simulink model "wec_reinforcementlearning"  (R2017b)
settings: Solver=VariableStepAuto  StartTime=0.0  StopTime=900  RelTol=1e-3
values from neighbouring files (symbols this model uses):
  B = zeros(vz,hz)    [ACTOR_CRITIC & SARSA.m]    (also in InputDataExtraction.m = 0.01; TDlearningExampleEforPosting.m)
  K = K_stiff*133333    (= 199999.5)    [InputDataExtraction.m]
  m = min(Out,[],2)    [ContinousControl.m]    (also in RL.m; RealTime_modif22.m)
undefined symbols (not defined in the file or in its folder): A, dzb_0, wp, zb_0
settings Model: Creator=brekken  LastModifiedBy=brekken
settings CodeAppCC: StateflowObjectComments=on

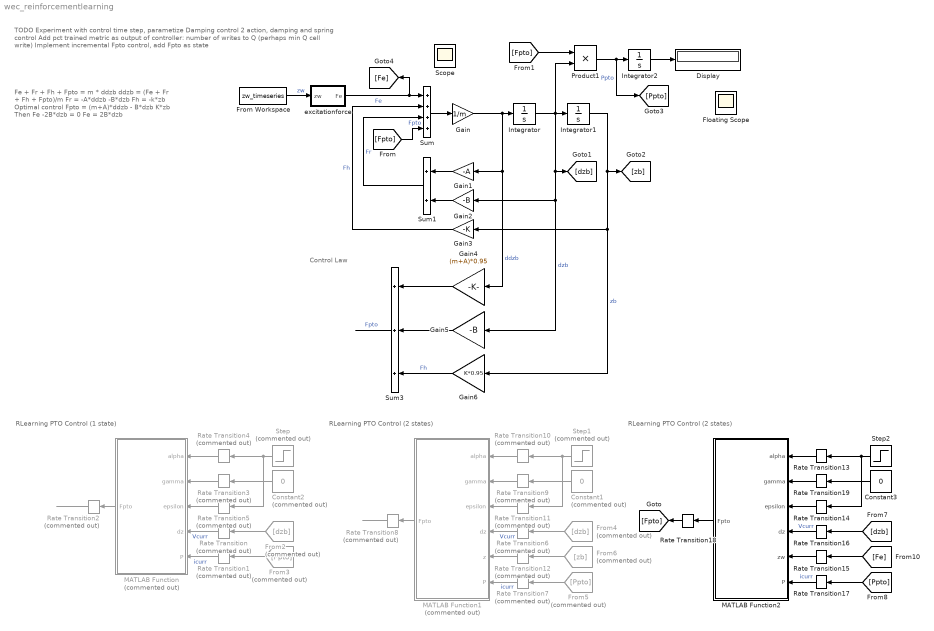
== system wec_reinforcementlearning ==
  note: Control Law
  note: TODO
      |
      | Experiment with control time step, parametize
      | Damping control
      | 2 action, damping and spring control
      | Add pct trained metric as output of controller: number of writes to Q (perhaps min Q cell write)
      | Implement incremental Fpto control, add Fpto as state
  note: RLearning PTO Control (1 state)
  note: Fe + Fr + Fh + Fpto = m * ddzb
      | ddzb = (Fe + Fr + Fh + Fpto)/m
      |
      | Fr = -A*ddzb -B*dzb
      |
      | Fh = -k*zb
      |
      | Optimal control
      | Fpto = (m+A)*ddzb - B*dzb K*zb
      | Then
      | Fe -2B*dzb = 0
      | Fe = 2B*dzb
  note: RLearning PTO Control (2 states)
  note: RLearning PTO Control (2 states)
  Constant1 : Constant  Commented=on  Value=0
  Constant2 : Constant  Commented=on  Value=0
  Constant3 : Constant  Value=0
  Display : Display
  Floating Scope : Scope
      settings: Floating=on
  From Workspace : FromWorkspace  VariableName=zw_timeseries  SampleTime=0  OutputAfterFinalValue=Setting to zero
  From2 : From  Commented=on  GotoTag=dzb
  From3 : From  Commented=on  GotoTag=Ppto
  From4 : From  Commented=on  GotoTag=dzb
  From5 : From  Commented=on  GotoTag=Ppto
  From6 : From  Commented=on  GotoTag=zb
  Gain : Gain  Gain=1/m
  Gain1 : Gain  Gain=-A
  Gain2 : Gain  Gain=-B
  Gain3 : Gain  Gain=-K
  Gain4 : Gain  Gain=(m+A)*0.95
  Gain5 : Gain  Gain=-B
  Gain6 : Gain  Gain=K*0.95
  Integrator : Integrator  InitialCondition=dzb_0
  Integrator1 : Integrator  InitialCondition=zb_0
  Integrator2 : Integrator
  MATLAB Function : MATLAB Function  Commented=on  TreatAsAtomicUnit=on
  MATLAB Function1 : MATLAB Function  Commented=on  TreatAsAtomicUnit=on
  MATLAB Function2 : MATLAB Function  TreatAsAtomicUnit=on
  Product1 : Product
  Rate Transition{,1,3..7,9..12} (11 alike) : RateTransition  Commented=on  Deterministic=off  OutPortSampleTime=0.1
  Rate Transition{13..17,19} (6 alike) : RateTransition  Deterministic=off  OutPortSampleTime=0.1
  Rate Transition18 : RateTransition  Deterministic=off  OutPortSampleTime=0
  Rate Transition2 : RateTransition  Commented=on  Deterministic=off  OutPortSampleTime=0
  Rate Transition8 : RateTransition  Commented=on  Deterministic=off  OutPortSampleTime=0
  Scope : Scope
  Step : Step  Commented=on  Time=700  Before=1  After=0  SampleTime=0
  Step1 : Step  Commented=on  Time=700  Before=1  After=0  SampleTime=0
  Step2 : Step  Time=800  Before=1  After=0  SampleTime=0
  Sum : Sum  Inputs=++++
  Sum1 : Sum
  Sum3 : Sum  Inputs=+++
  excitationforce : Subsystem
  wires:
  Gain/1 -> Gain1/1, Gain4/1, Integrator/1  "ddzb"
  Sum/1 -> Gain/1
  Sum1/1 -> Sum/3  "Fr"
  Gain3/1 -> Sum/2  "Fh"
  Gain1/1 -> Sum1/1
  Gain2/1 -> Sum1/2
  From Workspace/1 -> excitationforce/1(zw)  "zw"
  MATLAB Function/1(Fpto) -> Rate Transition2/1
  Rate Transition/1 -> MATLAB Function/4(dz)  "Vcurr"
  Rate Transition1/1 -> MATLAB Function/5(P)  "icurr"
  Rate Transition4/1 -> MATLAB Function/1(alpha)
  Rate Transition5/1 -> MATLAB Function/3(epsilon)
  Constant2/1 -> Rate Transition3/1
  Rate Transition3/1 -> MATLAB Function/2(gamma)
  Step/1 -> Rate Transition5/1, Rate Transition4/1
  Product1/1 -> [Ppto], Integrator2/1  "Ppto"
  Integrator2/1 -> Display/1
  [Fpto] -> Product1/1
  Rate Transition2/1 -> ?
  From2/1 -> Rate Transition/1
  From3/1 -> Rate Transition1/1
  Rate Transition6/1 -> MATLAB Function1/4(dz)  "Vcurr"
  Rate Transition7/1 -> MATLAB Function1/6(P)  "icurr"
  Rate Transition11/1 -> MATLAB Function1/3(epsilon)
  Rate Transition8/1 -> ?
  MATLAB Function1/1(Fpto) -> Rate Transition8/1
  Rate Transition10/1 -> MATLAB Function1/1(alpha)
  From4/1 -> Rate Transition6/1
  Constant1/1 -> Rate Transition9/1
  Rate Transition9/1 -> MATLAB Function1/2(gamma)
  From5/1 -> Rate Transition7/1
  Step1/1 -> Rate Transition11/1, Rate Transition10/1
  Rate Transition12/1 -> MATLAB Function1/5(z)
  From6/1 -> Rate Transition12/1
  excitationforce/1(Fe) -> [Fe], Sum/1  "Fe"
  Rate Transition17/1 -> MATLAB Function2/6(P)  "icurr"
  Constant3/1 -> Rate Transition19/1
  [Ppto] -> Rate Transition17/1
  Rate Transition14/1 -> MATLAB Function2/3(epsilon)
  Rate Transition13/1 -> MATLAB Function2/1(alpha)
  [dzb] -> Rate Transition16/1
  Rate Transition19/1 -> MATLAB Function2/2(gamma)
  Step2/1 -> Rate Transition14/1, Rate Transition13/1
  Rate Transition16/1 -> MATLAB Function2/4(dz)  "Vcurr"
  [Fe] -> Rate Transition15/1
  Rate Transition18/1 -> [Fpto]
  Rate Transition15/1 -> MATLAB Function2/5(zw)
  Integrator1/1 -> [zb], Gain6/1, Gain3/1  "zb"
  Gain5/1 -> Sum3/2
  Integrator/1 -> Product1/2, [dzb], Gain5/1, Gain2/1, Integrator1/1  "dzb"
  Gain4/1 -> Sum3/1
  Gain6/1 -> Sum3/3  "Fh"
  [Fpto] -> Sum/4  "Fpto"
  Sum3/1 -> ?  "Fpto"
  MATLAB Function2/1(Fpto) -> Rate Transition18/1

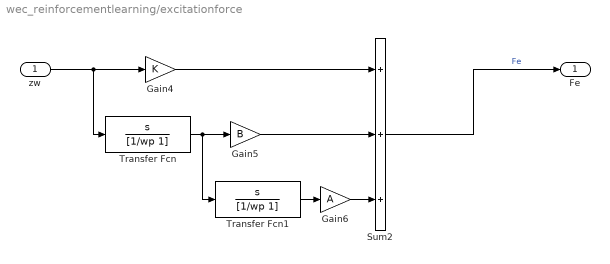
== system wec_reinforcementlearning/excitationforce ==
  zw : Inport
  Gain4 : Gain  Gain=K
  Gain5 : Gain  Gain=B
  Gain6 : Gain  Gain=A
  Sum2 : Sum  Inputs=+++
  Transfer Fcn : TransferFcn  Numerator=[1 0]  Denominator=[1/wp 1]
  Transfer Fcn1 : TransferFcn  Numerator=[1 0]  Denominator=[1/wp 1]
  Fe : Outport
  wires:
  Transfer Fcn/1 -> Transfer Fcn1/1, Gain5/1
  Gain5/1 -> Sum2/2
  Gain6/1 -> Sum2/3
  Sum2/1 -> Fe/1  "Fe"
  zw/1 -> Transfer Fcn/1, Gain4/1
  Transfer Fcn1/1 -> Gain6/1
  Gain4/1 -> Sum2/1

== matlab function wec_reinforcementlearning/MATLAB Function ==
  data: alpha input; gamma input; epsilon input; dz input; P input; Fpto output
function Fpto  = fcn(alpha,gamma,epsilon,dz,P)

% State and action binning
dzmin = -2;
dzmax = 2;
nstates = 20;
Fptomin = -1e6*0.1;
Fptomax = 1e6*0.1;
nactions = 20;

% Convert measurements to states
dzvec = linspace(dzmin,dzmax,nstates);
[~,st] = min(abs(dz - dzvec));

% Initialization for first time through
persistent Q c stm1 atm1
if isempty(Q)
    Q = rand(nstates,nactions);
end
if isempty(c)
    c = 1;
end 
if isempty(stm1)
    stm1 = 1;
end 
if isempty(atm1)
    atm1 = 1;
end 

% Reward
rt = P;

% Policy
% Choose the action associate with the highest value state
% with epsilon probability, choose at random
if rand > epsilon
    [~,at] = max(Q(st,:));
else
    at = randi([1 nactions]);
end

% Update knowledge
% Q(st,at) <- Q(st,at)*(1-alpha) + alpha*(rtp1 + gamma*Q(stp1,atp1))
% Q(stm1,atm1) <- Q(stm1,atm1)*(1-alpha) + alpha*(rt + gamma*Q(st,at))
Q(stm1,atm1) = Q(stm1,atm1)*(1-alpha) + alpha*(rt + gamma*Q(st,at));

% Convert action to output
Fptovec = linspace(Fptomin,Fptomax,nactions);
Fpto = Fptovec(at);

% Send data to next iteration
stm1 = st;
atm1 = at;
c = c+1;

== matlab function wec_reinforcementlearning/MATLAB Function1 ==
  data: alpha input; gamma input; epsilon input; dz input; z input; P input; Fpto output
function Fpto  = fcn(alpha,gamma,epsilon,dz,z,P)

% State and action binning
dzmin = -2;
dzmax = 2;
nstates1 = 20;
zmin = -2;
zmax = 2;
nstates2 = 20;
Fptomin = -1e6*0.1;
Fptomax = 1e6*0.1;
nactions = 20;

% Convert measurements to states
dzvec = linspace(dzmin,dzmax,nstates1);
[~,s1t] = min(abs(dz - dzvec));

% Convert measurements to states
zvec = linspace(zmin,zmax,nstates2);
[~,s2t] = min(abs(z - zvec));

% Initialization for first time through
persistent Q c s1tm1 s2tm1 atm1
if isempty(Q)
    Q = rand(nstates1,nstates2,nactions);
end
if isempty(c)
    c = 1;
end 
if isempty(s1tm1)
    s1tm1 = 1;
end 
if isempty(s2tm1)
    s2tm1 = 1;
end 
if isempty(atm1)
    atm1 = 1;
end 

% Reward
rt = P;

% Policy
% Choose the action associate with the highest value state
% with epsilon probability, choose at random
if rand > epsilon
    [~,at] = max(Q(s1t,s2t,:));
else
    at = randi([1 nactions]);
end

% Update knowledge
% Q(st,at) <- Q(st,at)*(1-alpha) + alpha*(rtp1 + gamma*Q(stp1,atp1))
% Q(stm1,atm1) <- Q(stm1,atm1)*(1-alpha) + alpha*(rt + gamma*Q(st,at))
Q(s1tm1,s2tm1,atm1) = Q(s1tm1,s2tm1,atm1)*(1-alpha) ...
    + alpha*(rt + gamma*Q(s1t,s2t,at));

% Convert action to output
Fptovec = linspace(Fptomin,Fptomax,nactions);
Fpto = Fptovec(at);

% Send data to next iteration
s1tm1 = s1t;
s2tm1 = s2t;
atm1 = at;
c = c+1;

== matlab function wec_reinforcementlearning/MATLAB Function2 ==
  data: alpha input; gamma input; epsilon input; dz input; zw input; P input; Fpto output
function Fpto  = fcn(alpha,gamma,epsilon,dz,zw,P)

% State and action binning
dzmin = -2;
dzmax = 2;
nstates1 = 20;
zwmin = -1e6;
zwmax = 1e6;
nstates2 = 20;
Fptomin = -1e6;
Fptomax = 1e6;
nactions = 20;

% Convert measurements to states
dzvec = linspace(dzmin,dzmax,nstates1);
[~,s1t] = min(abs(dz - dzvec));

% Convert measurements to states
zwvec = linspace(zwmin,zwmax,nstates2);
[~,s2t] = min(abs(zw - zwvec));

% Initialization for first time through
persistent Q c s1tm1 s2tm1 atm1
if isempty(Q)
    Q = rand(nstates1,nstates2,nactions);
end
if isempty(c)
    c = 1;
end 
if isempty(s1tm1)
    s1tm1 = 1;
end 
if isempty(s2tm1)
    s2tm1 = 1;
end 
if isempty(atm1)
    atm1 = 1;
end 

% Reward
rt = P;

% Policy
% Choose the action associate with the highest value state
% with epsilon probability, choose at random
if rand > epsilon
    [~,at] = max(Q(s1t,s2t,:));
else
    at = randi([1 nactions]);
end

% Update knowledge
% Q(st,at) <- Q(st,at)*(1-alpha) + alpha*(rtp1 + gamma*Q(stp1,atp1))
% Q(stm1,atm1) <- Q(stm1,atm1)*(1-alpha) + alpha*(rt + gamma*Q(st,at))
Q(s1tm1,s2tm1,atm1) = Q(s1tm1,s2tm1,atm1)*(1-alpha) ...
    + alpha*(rt + gamma*Q(s1t,s2t,at));

% Convert action to output
Fptovec = linspace(Fptomin,Fptomax,nactions);
Fpto = Fptovec(at);

% Send data to next iteration
s1tm1 = s1t;
s2tm1 = s2t;
atm1 = at;
c = c+1;
